simulink model "Model"  (Simulink 7.7)
settings: Solver=ode45  StartTime=0.0  StopTime=inf  FixedStep=0.01  RelTol=1e-3
values from neighbouring files (symbols this model uses):
  A = 0.1    [Model_param.m]
  B = 0.5    [Model_param.m]
  C = 100    [Model_param.m]
  C_R = 0    [Model_param.m]
  E0 = 10    [Model_param.m]
  J = 0.1    [Model_param.m]
  K = 0.00005    (= 5e-05)    [Model_param.m]
  Ke = 0.1    [Model_param.m]
  Km = 0.1    [Model_param.m]
  Lw = 0.1    [Model_param.m]
  Mobc = 0.1    [Model_param.m]
  Q = 1000    [Model_param.m]
  R_per = Period-1    (= 11)    [Model_param.m]
  R_ton = Period-Ton    (= 0)    [Model_param.m]
  Rw = 2    [Model_param.m]
  Smpl = 0.1    [Model_param.m]
  T = 1000    [Model_param.m]
libraries: simulink x1
settings Model: Creator=hp  LastModifiedBy=hp
settings RTWCC: CheckMdlBeforeBuild=Warning

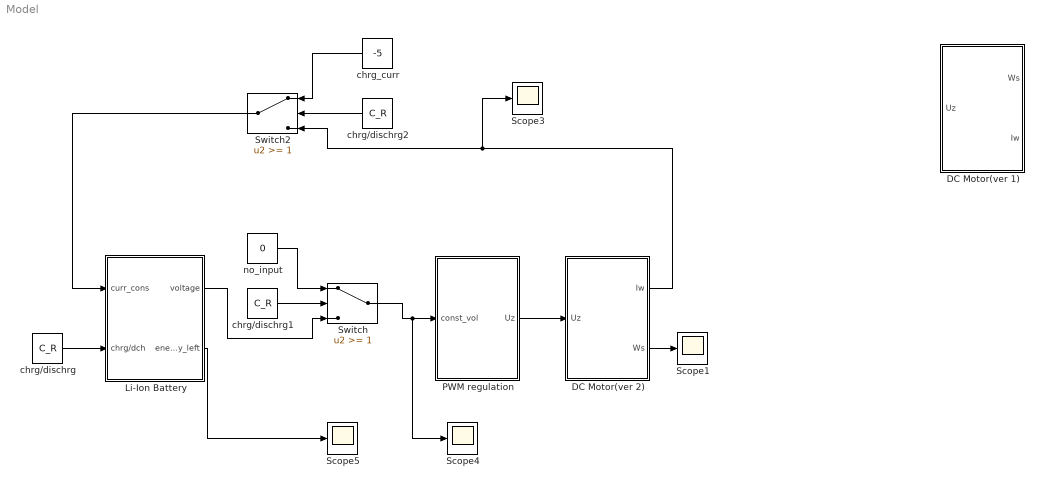
== system Model ==
  DC Motor(ver 1) : Subsystem
  DC Motor(ver 2) : Subsystem
  Li-Ion Battery : Subsystem
  PWM regulation : Subsystem
  Scope{1,3..5} (4 alike) : Scope
      Scope1 settings: YMin=-0.2  YMax=-0.2
      Scope3 settings: SaveName=ScopeData3
      Scope4 settings: YMin=-0.02  YMax=-0.02  SaveName=ScopeData4
      Scope5 settings: YMin=4.71698  YMax=5.2135
  Switch : Switch  Threshold=1  SampleTime=Smpl
  Switch2 : Switch  Threshold=1  SampleTime=Smpl
  chrg/dischrg : Constant  Value=C_R
  chrg/dischrg1 : Constant  Value=C_R
  chrg/dischrg2 : Constant  Value=C_R
  chrg_curr : Constant  Value=-5
  no_input : Constant  Value=0
  wires:
  chrg/dischrg/1 -> Li-Ion Battery/2(chrg/dch)
  DC Motor(ver 2)/2(Ws) -> Scope1/1
  DC Motor(ver 2)/1(Iw) -> Scope3/1, Switch2/3
  PWM regulation/1(Uz) -> DC Motor(ver 2)/1(Uz)
  Li-Ion Battery/2(energy_left) -> Scope5/1
  chrg/dischrg1/1 -> Switch/2
  Li-Ion Battery/1(voltage) -> Switch/3
  no_input/1 -> Switch/1
  Switch/1 -> PWM regulation/1(const_vol), Scope4/1
  chrg/dischrg2/1 -> Switch2/2
  chrg_curr/1 -> Switch2/1
  Switch2/1 -> Li-Ion Battery/1(curr_cons)

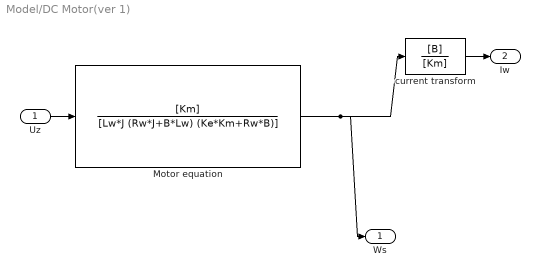
== system Model/DC Motor(ver 1) ==
  Uz : Inport
  Motor equation : TransferFcn  Numerator=[Km]  Denominator=[Lw*J (Rw*J+B*Lw) (Ke*Km+Rw*B)]
  current transform : TransferFcn  Numerator=[B]  Denominator=[Km]
  Ws : Outport
  Iw : Outport  Port=2
  wires:
  Motor equation/1 -> current transform/1, Ws/1
  current transform/1 -> Iw/1
  Uz/1 -> Motor equation/1

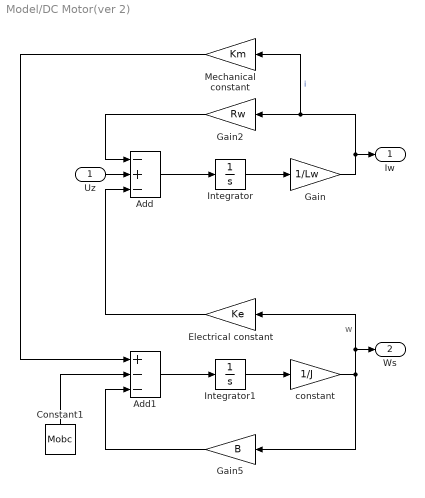
== system Model/DC Motor(ver 2) ==
  note: w
  Uz : Inport
  Add : Sum  Inputs=-+-
  Add1 : Sum  Inputs=+--
  Constant1 : Constant  Value=Mobc
  Electrical constant : Gain  Gain=Ke
  Gain : Gain  Gain=1/Lw
  Gain2 : Gain  Gain=Rw
  Gain5 : Gain  Gain=B
  Integrator : Integrator
  Integrator1 : Integrator
  Mechanical constant : Gain  Gain=Km
  constant : Gain  Gain=1/J
  Iw : Outport
  Ws : Outport  Port=2
  wires:
  Integrator1/1 -> constant/1
  Integrator/1 -> Gain/1
  Add/1 -> Integrator/1
  Add1/1 -> Integrator1/1
  constant/1 -> Gain5/1, Electrical constant/1, Ws/1
  Gain/1 -> Gain2/1, Mechanical constant/1, Iw/1  "i"
  Gain2/1 -> Add/1
  Electrical constant/1 -> Add/3
  Mechanical constant/1 -> Add1/1
  Gain5/1 -> Add1/3
  Constant1/1 -> Add1/2
  Uz/1 -> Add/2

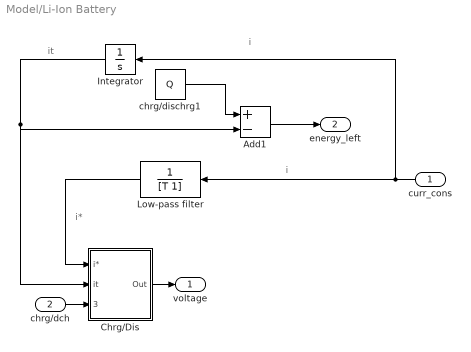
== system Model/Li-Ion Battery ==
  note: i
  note: it
  note: i*
  note: i
  curr_cons : Inport
  chrg/dch : Inport  Port=2
  Add1 : Sum  Inputs=+-
  Chrg/Dis : Subsystem
  Integrator : Integrator
  Low-pass filter : TransferFcn  Denominator=[T 1]
  chrg/dischrg1 : Constant  Value=Q
  voltage : Outport
  energy_left : Outport  Port=2
  wires:
  Integrator/1 -> Chrg/Dis/2(it), Add1/2
  Low-pass filter/1 -> Chrg/Dis/1(i*)
  curr_cons/1 -> Low-pass filter/1, Integrator/1
  Chrg/Dis/1(Out) -> voltage/1
  chrg/dch/1 -> Chrg/Dis/3(Chrg/Dis)
  chrg/dischrg1/1 -> Add1/1
  Add1/1 -> energy_left/1

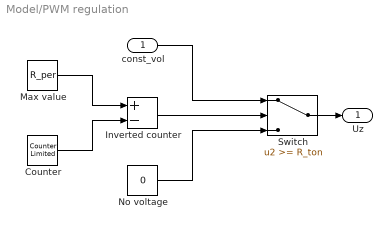
== system Model/PWM regulation ==
  const_vol : Inport
  Counter : simulink/Sources/Counter Limited  SystemSampleTime=-1  uplimit=R_per  tsamp=Smpl
  Inverted counter : Sum  Inputs=+-
  Max value : Constant  Value=R_per
  No voltage : Constant  Value=0
  Switch : Switch  Threshold=R_ton  SampleTime=Smpl
  Uz : Outport
  wires:
  No voltage/1 -> Switch/3
  Counter/1 -> Inverted counter/2
  Max value/1 -> Inverted counter/1
  Inverted counter/1 -> Switch/2
  const_vol/1 -> Switch/1
  Switch/1 -> Uz/1

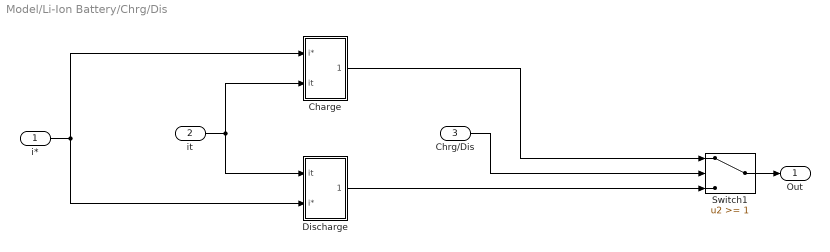
== system Model/Li-Ion Battery/Chrg/Dis ==
  i* : Inport
  it : Inport  Port=2
  Chrg/Dis : Inport  Port=3
  Charge : Subsystem
  Discharge : Subsystem
  Switch1 : Switch  Threshold=1
  Out : Outport
  wires:
  Charge/1(Out1) -> Switch1/1
  Discharge/1(Out1) -> Switch1/3
  it/1 -> Discharge/1(it), Charge/2(it)
  i*/1 -> Discharge/2(i*), Charge/1(i*)
  Switch1/1 -> Out/1
  Chrg/Dis/1 -> Switch1/2

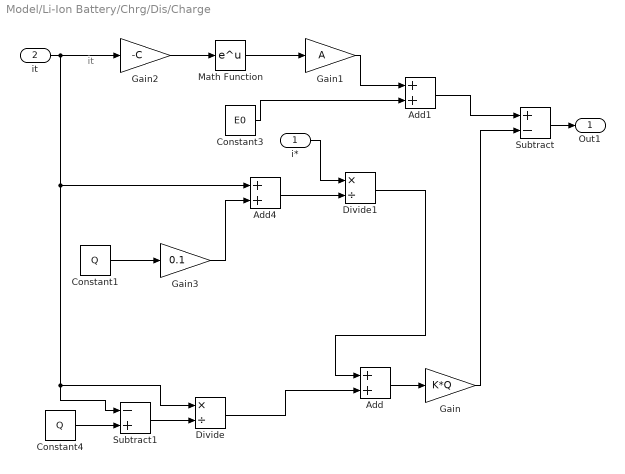
== system Model/Li-Ion Battery/Chrg/Dis/Charge ==
  note: it
  i* : Inport
  it : Inport  Port=2
  Add : Sum
  Add1 : Sum
  Add4 : Sum
  Constant1 : Constant  Value=Q
  Constant3 : Constant  Value=E0
  Constant4 : Constant  Value=Q
  Divide : Product  Inputs=*/
  Divide1 : Product  Inputs=*/
  Gain : Gain  Gain=K*Q
  Gain1 : Gain  Gain=A
  Gain2 : Gain  Gain=-C
  Gain3 : Gain  Gain=0.1
  Math Function : Math  SaturateOnIntegerOverflow=on
  Subtract : Sum  Inputs=+-
  Subtract1 : Sum  Inputs=-+
  Out1 : Outport
  wires:
  Subtract/1 -> Out1/1
  Subtract1/1 -> Divide/2
  it/1 -> Gain2/1, Subtract1/1, Divide/1, Add4/1
  Gain2/1 -> Math Function/1
  Math Function/1 -> Gain1/1
  Gain/1 -> Subtract/2
  Gain1/1 -> Add1/1
  Constant3/1 -> Add1/2
  Add1/1 -> Subtract/1
  Add/1 -> Gain/1
  Divide/1 -> Add/2
  Constant4/1 -> Subtract1/2
  Add4/1 -> Divide1/2
  Constant1/1 -> Gain3/1
  Gain3/1 -> Add4/2
  i*/1 -> Divide1/1
  Divide1/1 -> Add/1

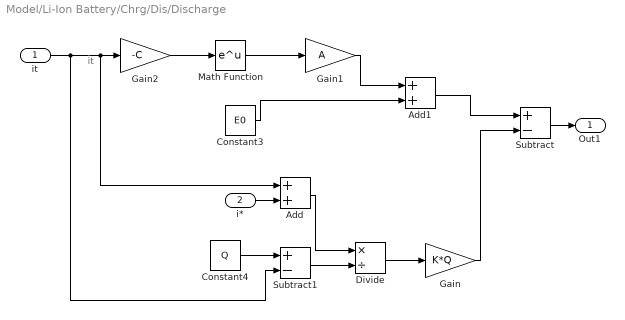
== system Model/Li-Ion Battery/Chrg/Dis/Discharge ==
  note: it
  it : Inport
  i* : Inport  Port=2
  Add : Sum
  Add1 : Sum
  Constant3 : Constant  Value=E0
  Constant4 : Constant  Value=Q
  Divide : Product  Inputs=*/
  Gain : Gain  Gain=K*Q
  Gain1 : Gain  Gain=A
  Gain2 : Gain  Gain=-C
  Math Function : Math  SaturateOnIntegerOverflow=on
  Subtract : Sum  Inputs=+-
  Subtract1 : Sum  Inputs=+-
  Out1 : Outport
  wires:
  Add1/1 -> Subtract/1
  Constant3/1 -> Add1/2
  Gain1/1 -> Add1/1
  Gain/1 -> Subtract/2
  Math Function/1 -> Gain1/1
  Gain2/1 -> Math Function/1
  it/1 -> Subtract1/2, Gain2/1, Add/1
  Constant4/1 -> Subtract1/1
  Subtract1/1 -> Divide/2
  Divide/1 -> Gain/1
  Add/1 -> Divide/1
  Subtract/1 -> Out1/1
  i*/1 -> Add/2
